simulink model "Copy_2_of_third_copy_of_Rotary_system_h_bridge_23a"  (R2023a)
settings: Solver=VariableStepAuto  StartTime=0.0  StopTime=0.15  FixedStep=1e-8  MaxStep=1e-7  RelTol=1e-6
InitFcn:
  | %% Parameters
  | 
  | param = struct();
  | 
  | % Volume of chambers
  | param.V1_0 = 1e-3;
  | param.V2_0 = 20e-6;
  | 
  | % Pressure rails
  | param.P_H = 20e6;
  | param.P_M = 10e6;
  | 
  | % Valve things
  | param.max_Avt = 0.5*0.25*pi*(20e-3)^2;
  | param.Cd = 0.6;
  | 
  | % Fluid properties
  | param.beta = 1.8e9;
  | param.rho = 870;
  | 
  | % Electric motor stuff
  | param.Kt = 70.5e-3;
  | param.Ke = 70.5e-3;
  | param.J_elec = 1530e-7;
  | 
  | % Pump things
  | param.J_hyd = 3000e-7;
  | param.hyd_D = 1.6e-6;    % In cc/rev
  | 
  | % Simulation time
  | T = 1;
  | param.on_time = 0;
  | 
  | % Piston parameters
  | param.A_cap = 0.0045;
values from neighbouring files (symbols this model uses):
  xdot = 1e-2    (= 0.01)    [Copy_2_of_PLOTS.m]    (also in PLOTS.m = 0.001)
settings Model: Creator=user  LastModifiedBy=ibrah408

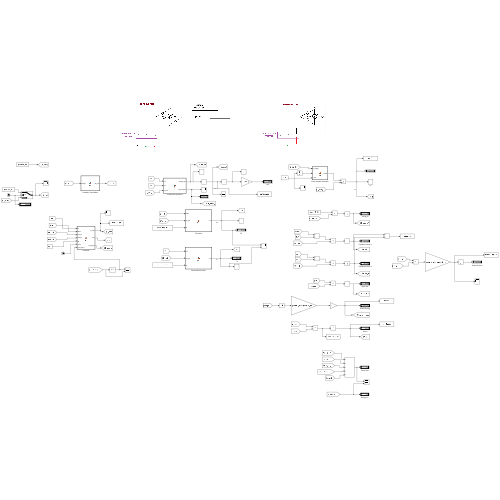
[thumbnail: Simulink's stored preview of the top-level diagram]
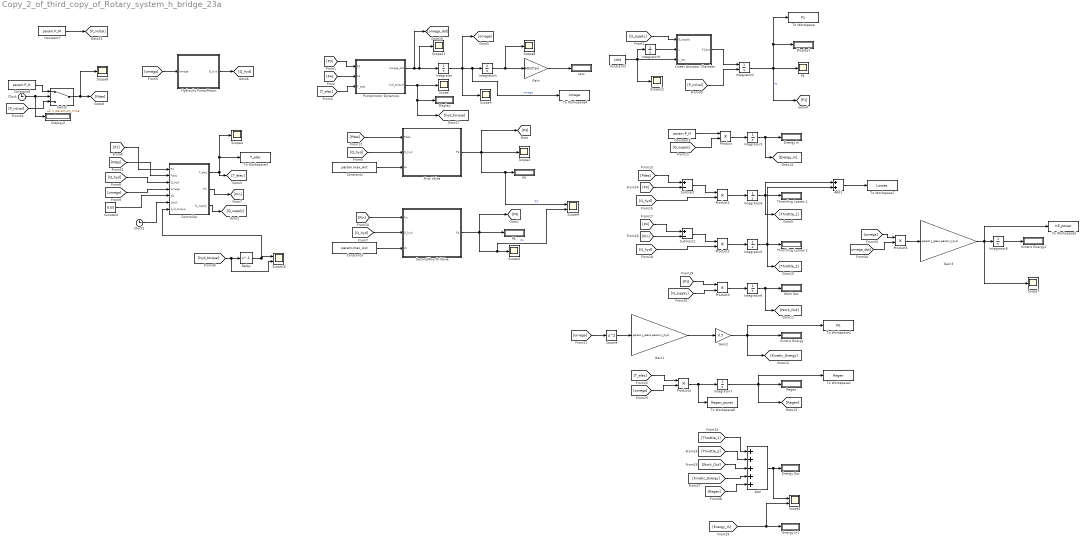
== system Copy_2_of_third_copy_of_Rotary_system_h_bridge_23a ==
  Add : Sum  Inputs=+++++
  Add1 : Sum
  Clock : Clock
  Clock1 : Clock
  Constant : Constant  Value=0.05
  Constant1 : Constant  Value=xdot
  Constant2 : Constant  Value=param.max_Avt
  Constant3 : Constant  Value=param.max_Avt
  Constant5 : Constant  Value=param.P_H
  Constant6 : Constant  Value=param.P_H
  Constant7 : Constant  Value=param.P_M
  Controller : MATLAB Function  TreatAsAtomicUnit=on
  Delay : Delay  DelayLength=1
  Display : Display
  Display1 : Display
  Display2 : Display
  Energy In : Display
  Energy In1 : Display
  Energy Out : Display
  First Valve : MATLAB Function  TreatAsAtomicUnit=on
  Gain : Gain  Gain=60/(2*pi)
  Gain1 : Gain  Gain=param.J_elec+param.J_hyd
  Gain2 : Gain  Gain=0.5
  Gain3 : Gain  Gain=param.J_elec+param.J_hyd
  Hydraulic Pump/Motor : MATLAB Function  TreatAsAtomicUnit=on
  Integrator{,1,3..9} (9 alike) : Integrator
  Integrator2 : Integrator  InitialConditionSource=external  InitialCondition=param.P_M
  Kinetic Energy : Display
  Kinetic Energy1 : Display
  Linear Actuator Chamber : MATLAB Function  TreatAsAtomicUnit=on
  P1 : Scope
  P3 : Display
  P4 : Display
  Product{,1..5} (6 alike) : Product
  Pump/motor Dynamics : MATLAB Function  TreatAsAtomicUnit=on
  Regen : Display
  Scope{,2..8,11..12} (10 alike) : Scope
  Scope1 : Scope  NumInputPorts=2
  Scope10 : Scope  NumInputPorts=2
  Scope9 : Scope  NumInputPorts=2
  Second/Fourth Valve : MATLAB Function  TreatAsAtomicUnit=on
  Square : Math  Operator=square
  Subtract : Sum  Inputs=+-
  Subtract1 : Sum  Inputs=+-
  Switch : Switch  Criteria=u2 > Threshold  Threshold=param.on_time  SaturateOnIntegerOverflow=off  InputSameDT=off
  Throttling Losses 1 : Display
  Throttling Losses 2 : Display
  To Workspace : ToWorkspace  VariableName=P1  SaveFormat=Timeseries  SampleTime=-1
  To Workspace1 : ToWorkspace  VariableName=Regen  SaveFormat=Timeseries  SampleTime=-1
  To Workspace2 : ToWorkspace  VariableName=KE  SaveFormat=Timeseries  SampleTime=-1
  To Workspace3 : ToWorkspace  VariableName=T_elec  SaveFormat=Timeseries  SampleTime=-1
  To Workspace4 : ToWorkspace  VariableName=omega  SaveFormat=Timeseries  SampleTime=-1
  To Workspace5 : ToWorkspace  VariableName=KE_power  SaveFormat=Timeseries  SampleTime=-1
  To Workspace6 : ToWorkspace  VariableName=Regen_power  SaveFormat=Timeseries  SampleTime=-1
  To Workspace7 : ToWorkspace  VariableName=Losses  SaveFormat=Timeseries  SampleTime=-1
  Work Out : Display
  revs : Display
  wires:
  Pump/motor Dynamics/1(omega_dot) -> [omega_dot], Scope11/1, Integrator/1
  Integrator/1 -> Scope5/1, [omega], To Workspace4/1, Integrator1/1  "omega"
  Integrator1/1 -> Scope8/1, Gain/1
  Gain/1 -> revs/1
  Constant2/1 -> First Valve/3(Av)
  Constant3/1 -> Second/Fourth Valve/3(Av)
  Linear Actuator Chamber/1(P1dot) -> Integrator2/1
  Integrator2/1 -> [P1], To Workspace/1, Display1/1, P1/1  "P1"
  First Valve/1(P3) -> Scope2/1, [P3], Scope9/1, P3/1  "P3"
  Second/Fourth Valve/1(P4) -> Scope9/2, Scope3/1, [P4], P4/1  "P4"
  Constant/1 -> Controller/5(Kd)
  [P4] -> Pump/motor Dynamics/2(P4)
  [P3] -> Pump/motor Dynamics/1(P3)
  [Pdes] -> First Valve/1(Pdes)
  Controller/3(Q_supply) -> [Q_supply]
  [Q_supply] -> Linear Actuator Chamber/1(Q_supply)
  Controller/1(T_elec) -> To Workspace3/1, Scope4/1, [T_elec]
  [T_elec] -> Pump/motor Dynamics/3(T_elec)
  [P1] -> Controller/1(P1)
  [Pdes] -> Controller/2(Pdes)
  [omega] -> Hydraulic Pump/Motor/1(omega)
  Hydraulic Pump/Motor/1(Q_hyd) -> [Q_hyd]
  [Q_hyd] -> First Valve/2(Q_hyd)
  [Q_hyd] -> Second/Fourth Valve/2(Q_hyd)
  [Q_hyd] -> Controller/3(Q_hyd)
  [omega] -> Controller/4(omega)
  Controller/2(Pin) -> [Pin]
  [Pin] -> Second/Fourth Valve/1(Pin)
  [Q_supply] -> Product/2
  Constant5/1 -> Product/1
  Product/1 -> Integrator3/1
  Integrator3/1 -> [Energy_In], Energy In/1
  Subtract/1 -> Product1/1
  [Pdes] -> Subtract/1
  [P3] -> Subtract/2
  [Q_hyd] -> Product1/2
  Product1/1 -> Integrator4/1
  Product2/1 -> Integrator5/1
  [Q_hyd] -> Product2/2
  Subtract1/1 -> Product2/1
  Integrator5/1 -> Add1/2, [Throttle_2], Throttling Losses 2/1
  [P4] -> Subtract1/1
  [Pin] -> Subtract1/2
  [Q_supply] -> Product3/2
  [P1] -> Product3/1
  Product3/1 -> Integrator6/1
  Integrator6/1 -> [Work_Out], Work Out/1
  [omega] -> Square/1
  Square/1 -> Gain1/1
  Gain1/1 -> Gain2/1
  Gain2/1 -> To Workspace2/1, Kinetic Energy/1, [Kinetic_Energy]
  Pump/motor Dynamics/2(hyd_torque) -> [hyd_torque], Display/1, Scope/1
  [T_elec] -> Product4/1
  [omega] -> Product4/2
  Product4/1 -> To Workspace6/1, Integrator7/1
  Integrator7/1 -> To Workspace1/1, [Regen], Regen/1
  Integrator4/1 -> Add1/1, [Throttle_1], Throttling Losses 1/1
  [Throttle_1] -> Add/1
  [Throttle_2] -> Add/2
  [Work_Out] -> Add/3
  [Kinetic_Energy] -> Add/4
  [Regen] -> Add/5
  Add/1 -> Scope1/1, Energy Out/1
  [Energy_In] -> Scope1/2, Energy In1/1
  [P_initial] -> Integrator2/2
  Constant7/1 -> [P_initial]
  Clock/1 -> Display2/1, Switch/2
  Constant6/1 -> Switch/1
  [P_initial] -> Switch/3
  Switch/1 -> Scope6/1, [Pdes]
  Clock1/1 -> Controller/6(clock)
  [omega] -> Product5/1
  [omega_dot] -> Product5/2
  Product5/1 -> Gain3/1
  Gain3/1 -> Integrator8/1, To Workspace5/1, Scope7/1
  Integrator8/1 -> Kinetic Energy1/1
  Add1/1 -> To Workspace7/1
  [hyd_torque] -> Scope10/2, Delay/1
  Delay/1 -> Controller/7(hyd_torque), Scope10/1
  Constant1/1 -> Scope12/1, Integrator9/1, Linear Actuator Chamber/3(x_dot)
  Integrator9/1 -> Linear Actuator Chamber/2(x)

== matlab function Copy_2_of_third_copy_of_Rotary_system_h_bridge_23a/Pump//motor Dynamics ==
  data: omega_dot output; P3 input; P4 input; param parameter; T_elec input; hyd_torque output
function [omega_dot, hyd_torque] = fcn(P3, P4, param, T_elec)

hyd_torque = (param.hyd_D/(2*pi))*(P3-P4);
omega_dot = (1/(param.J_elec+param.J_hyd))*(hyd_torque - T_elec);

== matlab function Copy_2_of_third_copy_of_Rotary_system_h_bridge_23a/Hydraulic Pump//Motor ==
  data: Q_hyd output; omega input; param parameter
function Q_hyd   = fcn(omega, param)

Q_hyd = (param.hyd_D/(2*pi))*omega;

== matlab function Copy_2_of_third_copy_of_Rotary_system_h_bridge_23a/First Valve ==
  data: Pdes input; P3 output; Q_hyd input; Av input; param parameter
function P3 = fcn(Pdes, Q_hyd, Av, param)

K = param.Cd*Av*sqrt(2/param.rho);

P3 = Pdes - (Q_hyd/K)^2;

== matlab function Copy_2_of_third_copy_of_Rotary_system_h_bridge_23a/Second//Fourth Valve ==
  data: Pin input; P4 output; Q_hyd input; Av input; param parameter
function P4 = fcn(Pin, Q_hyd, Av, param)

K = param.Cd*Av*sqrt(2/param.rho);
P4 = Pin + (Q_hyd/K)^2;

== matlab function Copy_2_of_third_copy_of_Rotary_system_h_bridge_23a/Linear Actuator Chamber ==
  data: P1dot output; Q_supply input; param parameter; x input; x_dot input
function P1dot = fcn(Q_supply, param, x, x_dot)

P1dot = (param.beta/(param.V1_0+param.A_cap*x))*(Q_supply - param.A_cap*x_dot);

== matlab function Copy_2_of_third_copy_of_Rotary_system_h_bridge_23a/Controller ==
  data: P1 input; Pdes input; Q_hyd input; omega input; Kd input; clock input; param parameter; T_elec output; Pin output; Q_supply output; hyd_torque input
function [T_elec, Pin, Q_supply] = fcn(P1, Pdes, Q_hyd, omega, Kd, clock, param, hyd_torque)

if clock > param.on_time
    if abs(P1-Pdes)<1e4
        if omega < 1
            T_elec = Kd*omega;
            Pin = Pdes;
            Q_supply = 0;
        else
            T_elec = 30;
            Pin = Pdes;
            Q_supply = 0;
        end
    else
        if omega >= 300
            T_elec = hyd_torque;
            Pin = P1;
            Q_supply = Q_hyd;
        else
            T_elec = -30;
            Pin = P1;
            Q_supply = Q_hyd;
        end
    end
else
    T_elec = 0;
    Pin = Pdes;
    Q_supply = 0;
end
